simulink model "MPC_Kalman"  (R2015a)
settings: Solver=ode4  StartTime=0.0  StopTime=10  FixedStep=0.01  RelTol=1e-3
values from neighbouring files (symbols this model uses):
  delay_time = 0    [MPC-PID-Data-0ms.mat]    (also in MPC-PID-Data-150ms.mat = 0.15; MPC-PID-Data-250ms.mat = 0.25; MPC-PID-Data-50ms.mat = 0.05)
libraries: simulink x8
settings Model: Creator=LAB425  LastModifiedBy=LAB425

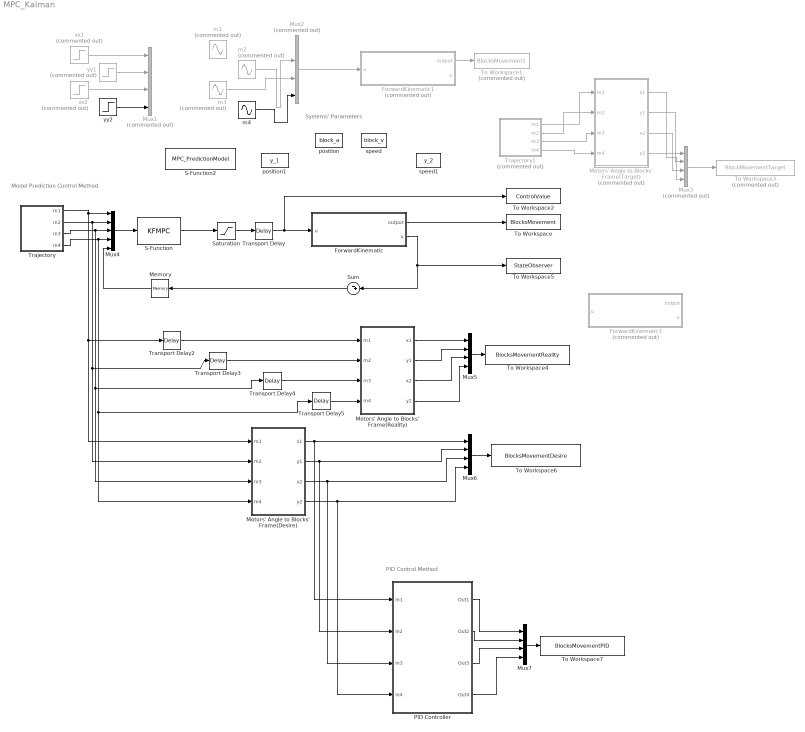
== system MPC_Kalman ==
  note: PID Control Method
  note: Model Prediction Control Method
  note: Systems' Parameters
  ForwardKinematic : MATLAB Function  TreatAsAtomicUnit=on
  ForwardKinematic1 : MATLAB Function  Commented=on  TreatAsAtomicUnit=on
  ForwardKinematic3 : MATLAB Function  Commented=on  TreatAsAtomicUnit=on
  Memory : Memory  X0=[0,0,0,0,0,0,0,0]
  Motors' Angle to Blocks' Frame(Desire) : MATLAB Function  TreatAsAtomicUnit=on
  Motors' Angle to Blocks' Frame(Reality) : MATLAB Function  TreatAsAtomicUnit=on
  "Motors' Angle to Blocks' Frame(Target) " : MATLAB Function  Commented=on  TreatAsAtomicUnit=on
  Mux1 : Mux  Commented=on
  Mux2 : Mux  Commented=on
  Mux3 : Mux  Commented=on
  Mux4 : Mux  Inputs=5
  Mux5 : Mux
  Mux6 : Mux
  Mux7 : Mux
  PID Controller : Subsystem
  S-Function : S-Function  FunctionName=KFMPC
  S-Function2 : S-Function  FunctionName=MPC_PredictionModel
  Saturation : Saturate  UpperLimit=1  LowerLimit=-1
  Sum : Sum  Inputs=-+|
  To Workspace : ToWorkspace  VariableName=BlocksMovement  SaveFormat=Timeseries  SampleTime=-1
  To Workspace1 : ToWorkspace  Commented=on  VariableName=BlocksMovement1  SaveFormat=Timeseries  SampleTime=-1
  To Workspace2 : ToWorkspace  VariableName=ControlValue  SaveFormat=Timeseries  SampleTime=-1
  To Workspace3 : ToWorkspace  Commented=on  VariableName=BlockMovementTarget  SaveFormat=Timeseries  SampleTime=-1
  To Workspace4 : ToWorkspace  VariableName=BlocksMovementReality  SaveFormat=Timeseries  SampleTime=-1
  To Workspace5 : ToWorkspace  VariableName=StateObserver  SaveFormat=Timeseries  SampleTime=-1
  To Workspace6 : ToWorkspace  VariableName=BlocksMovementDesire  SaveFormat=Timeseries  SampleTime=-1
  To Workspace7 : ToWorkspace  VariableName=BlocksMovementPID  SaveFormat=Timeseries  SampleTime=-1
  Trajectory : Subsystem
  Trajectory1 : Subsystem  Commented=on
  Transport Delay{,2..5} (5 alike) : TransportDelay  DelayTime=delay_time
  m1 : Sin  Commented=on  SampleTime=0
  m2 : Sin  Commented=on  Frequency=2  SampleTime=0
  m3 : Sin  Commented=on  Phase=3.14  SampleTime=0
  m4 : Sin  Frequency=2  Phase=3.14  SampleTime=0
  position : DataStoreMemory  DataStoreName=block_a  ReadBeforeWriteMsg=warning  WriteAfterWriteMsg=warning  WriteAfterReadMsg=warning  InitialValue=[0,0,0,0]  OutDataTypeStr=double
  position1 : DataStoreMemory  DataStoreName=y_1  ReadBeforeWriteMsg=warning  WriteAfterWriteMsg=warning  WriteAfterReadMsg=warning  InitialValue=[0,0,0,0]  OutDataTypeStr=double
  speed : DataStoreMemory  DataStoreName=block_v  ReadBeforeWriteMsg=warning  WriteAfterWriteMsg=warning  WriteAfterReadMsg=warning  InitialValue=[0,0,0,0]  OutDataTypeStr=double
  speed1 : DataStoreMemory  DataStoreName=y_2  ReadBeforeWriteMsg=warning  WriteAfterWriteMsg=warning  WriteAfterReadMsg=warning  InitialValue=[0,0,0,0]  OutDataTypeStr=double
  xx1 : Step  Commented=on  Time=0  Before=-2  After=-2
  xx2 : Step  Commented=on  Time=0  Before=0.5  After=0.5
  yy1 : Step  Commented=on  Time=0  Before=-2  After=-2
  yy2 : Step  Time=5  Before=1
  wires:
  xx1/1 -> Mux1/1
  yy2/1 -> Mux1/4
  yy1/1 -> Mux1/2
  xx2/1 -> Mux1/3
  m2/1 -> Mux2/2
  m3/1 -> Mux2/3
  m4/1 -> Mux2/4
  Mux2/1 -> ForwardKinematic1/1(u)
  ForwardKinematic1/1(output) -> To Workspace1/1
  Mux4/1 -> S-Function/1
  Memory/1 -> Mux4/5
  S-Function/1 -> Saturation/1
  Trajectory/1(m1) -> Motors' Angle to Blocks' Frame(Desire)/1(m1), Transport Delay2/1, Mux4/1
  Trajectory/3(m3) -> Motors' Angle to Blocks' Frame(Desire)/3(m3), Transport Delay4/1, Mux4/3
  Trajectory1/1(m1) -> "Motors' Angle to Blocks' Frame(Target) "/1(m1)
  Trajectory1/2(m2) -> "Motors' Angle to Blocks' Frame(Target) "/2(m2)
  Trajectory1/3(m3) -> "Motors' Angle to Blocks' Frame(Target) "/3(m3)
  Trajectory1/4(m4) -> "Motors' Angle to Blocks' Frame(Target) "/4(m4)
  Mux3/1 -> To Workspace3/1
  "Motors' Angle to Blocks' Frame(Target) "/1(x1) -> Mux3/1
  "Motors' Angle to Blocks' Frame(Target) "/2(y1) -> Mux3/2
  "Motors' Angle to Blocks' Frame(Target) "/3(x2) -> Mux3/3
  "Motors' Angle to Blocks' Frame(Target) "/4(y2) -> Mux3/4
  Trajectory/4(m4) -> Motors' Angle to Blocks' Frame(Desire)/4(m4), Transport Delay5/1, Mux4/4
  Motors' Angle to Blocks' Frame(Reality)/1(x1) -> Mux5/1
  Motors' Angle to Blocks' Frame(Reality)/2(y1) -> Mux5/2
  Motors' Angle to Blocks' Frame(Reality)/3(x2) -> Mux5/3
  Motors' Angle to Blocks' Frame(Reality)/4(y2) -> Mux5/4
  Mux5/1 -> To Workspace4/1
  Saturation/1 -> Transport Delay/1
  Sum/1 -> Memory/1
  Transport Delay2/1 -> Motors' Angle to Blocks' Frame(Reality)/1(m1)
  Transport Delay3/1 -> Motors' Angle to Blocks' Frame(Reality)/2(m2)
  Transport Delay4/1 -> Motors' Angle to Blocks' Frame(Reality)/3(m3)
  Transport Delay5/1 -> Motors' Angle to Blocks' Frame(Reality)/4(m4)
  ForwardKinematic/2(x) -> Sum/2, To Workspace5/1
  ForwardKinematic/1(output) -> To Workspace/1
  Transport Delay/1 -> ForwardKinematic/1(u), To Workspace2/1
  Mux6/1 -> To Workspace6/1
  Trajectory/2(m2) -> Motors' Angle to Blocks' Frame(Desire)/2(m2), Transport Delay3/1, Mux4/2
  Motors' Angle to Blocks' Frame(Desire)/1(x1) -> Mux6/1, PID Controller/1(in1)
  Motors' Angle to Blocks' Frame(Desire)/2(y1) -> Mux6/2, PID Controller/2(In2)
  Mux7/1 -> To Workspace7/1
  Motors' Angle to Blocks' Frame(Desire)/3(x2) -> Mux6/3, PID Controller/3(In3)
  Motors' Angle to Blocks' Frame(Desire)/4(y2) -> PID Controller/4(In4), Mux6/4
  PID Controller/1(Out1) -> Mux7/1
  PID Controller/2(Out2) -> Mux7/2
  PID Controller/3(Out3) -> Mux7/3
  PID Controller/4(Out4) -> Mux7/4

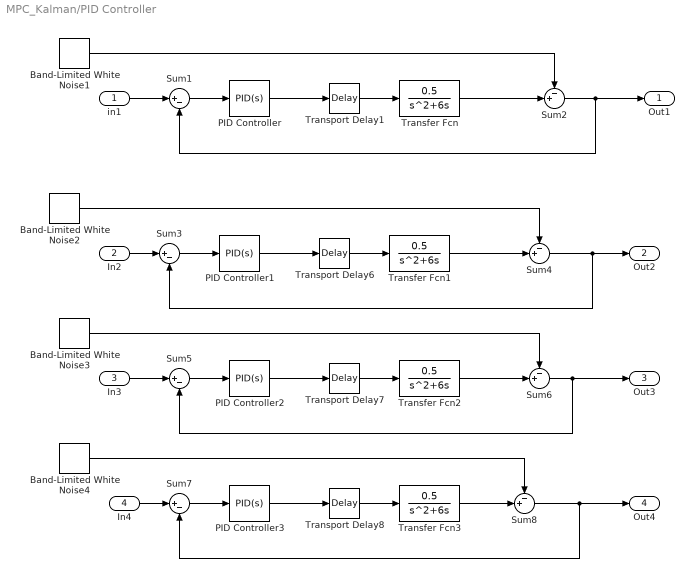
== system MPC_Kalman/PID Controller ==
  in1 : Inport
  In2 : Inport  Port=2
  In3 : Inport  Port=3
  In4 : Inport  Port=4
  Band-Limited White Noise{1..4} (4 alike) : simulink/Sources/Band-Limited White Noise  Cov=[0.00001]  Ts=0.01  seed=[23341]
  PID Controller{,1..3} (4 alike) : simulink/Continuous/PID Controller  Controller=PID  TimeDomain=Continuous-time  SampleTime=-1  IntegratorMethod=Forward Euler  FilterMethod=Forward Euler  Form=Parallel  UseFilter=on  ControllerParametersSource=internal  P=60  I=2  D=0  N=100  InitialConditionSource=internal  InitialConditionForIntegrator=0  InitialConditionForFilter=0  ExternalReset=none  LimitOutput=off  UpperSaturationLimit=inf  LowerSaturationLimit=-inf  LinearizeAsGain=on  AntiWindupMode=none  Kb=1  TrackingMode=off  Kt=1  PParamMin=[]  PParamMax=[]  IParamMin=[]  IParamMax=[]  DParamMin=[]  DParamMax=[]  NParamMin=[]  NParamMax=[]  KbParamMin=[]  KbParamMax=[]  KtParamMin=[]  KtParamMax=[]  POutMin=[]  POutMax=[]  IOutMin=[]  IOutMax=[]  DOutMin=[]  DOutMax=[]  NOutMin=[]  NOutMax=[]  KbOutMin=[]  KbOutMax=[]  KtOutMin=[]  KtOutMax=[]  IntegratorOutMin=[]  IntegratorOutMax=[]  FilterOutMin=[]  FilterOutMax=[]  SumOutMin=[]  SumOutMax=[]  SumI1OutMin=[]  SumI1OutMax=[]  SumI2OutMin=[]  SumI2OutMax=[]  SumI3OutMin=[]  SumI3OutMax=[]  SumDOutMin=[]  SumDOutMax=[]  SaturationOutMin=[]  SaturationOutMax=[]  IntegratorContinuousStateAttributes=''  IntegratorStateMustResolveToSignalObject=off  IntegratorRTWStateStorageClass=Auto  FilterContinuousStateAttributes=''  FilterStateMustResolveToSignalObject=off  FilterRTWStateStorageClass=Auto  DifferentiatorICPrevScaledInput=0  DifferentiatorOutMin=[]  DifferentiatorOutMax=[]
  Sum{1,3,5,7} (4 alike) : Sum  Inputs=|+-
  Sum{2,4,6,8} (4 alike) : Sum  Inputs=-+|
  Transfer Fcn{,1..3} (4 alike) : TransferFcn  Numerator=[0.5]  Denominator=[1 6 0]
  Transport Delay{1,6..8} (4 alike) : TransportDelay  DelayTime=delay_time
  Out1 : Outport
  Out2 : Outport  Port=2
  Out3 : Outport  Port=3
  Out4 : Outport  Port=4
  wires:
  Transport Delay1/1 -> Transfer Fcn/1
  PID Controller/1 -> Transport Delay1/1
  Sum1/1 -> PID Controller/1
  PID Controller2/1 -> Transport Delay7/1
  Transfer Fcn2/1 -> Sum6/2
  Sum5/1 -> PID Controller2/1
  Band-Limited White Noise3/1 -> Sum6/1
  Transport Delay7/1 -> Transfer Fcn2/1
  Transport Delay6/1 -> Transfer Fcn1/1
  Sum3/1 -> PID Controller1/1
  Transfer Fcn1/1 -> Sum4/2
  Band-Limited White Noise2/1 -> Sum4/1
  PID Controller1/1 -> Transport Delay6/1
  Sum2/1 -> Sum1/2, Out1/1
  Sum6/1 -> Sum5/2, Out3/1
  In2/1 -> Sum3/1
  Sum8/1 -> Sum7/2, Out4/1
  in1/1 -> Sum1/1
  In4/1 -> Sum7/1
  In3/1 -> Sum5/1
  PID Controller3/1 -> Transport Delay8/1
  Transfer Fcn3/1 -> Sum8/2
  Sum7/1 -> PID Controller3/1
  Band-Limited White Noise4/1 -> Sum8/1
  Transport Delay8/1 -> Transfer Fcn3/1
  Band-Limited White Noise1/1 -> Sum2/1
  Transfer Fcn/1 -> Sum2/2
  Sum4/1 -> Sum3/2, Out2/1

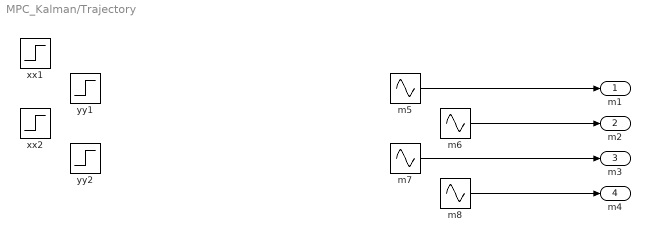
== system MPC_Kalman/Trajectory ==
  m5 : Sin  SampleTime=0
  m6 : Sin  Frequency=2  SampleTime=0
  m7 : Sin  Phase=3.14  SampleTime=0
  m8 : Sin  Frequency=2  Phase=3.14  SampleTime=0
  xx1 : Step
  xx2 : Step  After=-1
  yy1 : Step
  yy2 : Step  After=-1
  m1 : Outport
  m2 : Outport  Port=2
  m3 : Outport  Port=3
  m4 : Outport  Port=4
  wires:
  m6/1 -> m2/1
  m5/1 -> m1/1
  m7/1 -> m3/1
  m8/1 -> m4/1

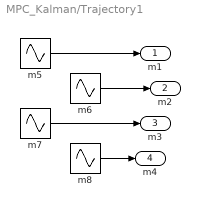
== system MPC_Kalman/Trajectory1 ==
  m5 : Sin  SampleTime=0
  m6 : Sin  Frequency=2  SampleTime=0
  m7 : Sin  Phase=3.14  SampleTime=0
  m8 : Sin  Frequency=2  Phase=3.14  SampleTime=0
  m1 : Outport
  m2 : Outport  Port=2
  m3 : Outport  Port=3
  m4 : Outport  Port=4
  wires:
  m6/1 -> m2/1
  m5/1 -> m1/1
  m7/1 -> m3/1
  m8/1 -> m4/1

== matlab function MPC_Kalman/ForwardKinematic1 ==
  data: output output; u input; block_v data_store_memory; block_a data_store_memory; x output
function [output,x] = RobotForwardKinematic(u) %输入1x4
global block_v block_a 
%block_v：上一时刻的角速度
%block_a：上一时刻的角度
%% 单电机状态方程
A = [0 1 0 0 0 0 0 0;
     0.005 0.045 0 0 0 0 0 0;
     0 0 0 1 0 0 0 0;
     0 0 0.0185 0.0251 0 0 0 0;
     0 0 0 0 0 1 0 0;
     0 0 0 0 0.0065 -0.0258 0 0;
     0 0 0 0 0 0 0 1;
     0 0 0 0 0 0 -0.023 0.0084]; 
b = [0 0 0 0;
     1.8899 0 0 0;
     0 0 0 0;
     0 1.8777 0 0;
     0 0 0 0;
     0 0 1.7655 0;
     0 0 0 0;
     0 0 0 1.7735];
C = [0 1 0 0 0 0 0 0;
     0 0 0 1 0 0 0 0;
     0 0 0 0 0 1 0 0;
     0 0 0 0 0 0 0 1];
% X = [0,1;-a2,-a1];
% H = [0,b]';
% C = [0,1];
delta_u = u - block_a;
v = delta_u ./ 0.01;
a = (v - block_v) ./ 0.01;
block_v = v;
block_a = u;
x = [v(1);a(1);v(2);a(2);v(3);a(3);v(4);a(4)];
output = C * (A * x + b * u);
%%

== matlab function MPC_Kalman/Motors' Angle to Blocks' Frame(Reality) ==
  data: x1 output; m1 input; y1 output; x2 output; m2 input; m3 input; m4 input; y2 output
function [x1,y1,x2,y2] = Signal(m1,m2,m3,m4)



%m1,m2,m3,m4为四个电机的当前时刻的角度值

%最远距离
D = 1.8;
% %螺距
% n = 0.02;
% %最大圈数
% ratio = D / n;
v=sqrt(0.01)*randn(4,1);
x1 = m1 * D + v(1);
y1 = m2 * D + v(2);
x2 = m3 * D + v(3);
y2 = m4 * D + v(4);

if x1>=2
    x1=2;
else
    if x1<=-2
        x1=-2;
    end
end
if x2>=2
    x2=2;
else
    if x2<=-2
        x2=-2;
    end
end
if y1>=2
    y1=2;
else
    if y1<=-2
        y1=-2;
    end
end
if y2>=2
    y2=2;
else
    if y2<=-2
        y2=-2;
    end
end

== matlab function MPC_Kalman/Motors' Angle to Blocks' Frame(Desire) ==
  data: x1 output; m1 input; y1 output; x2 output; m2 input; m3 input; m4 input; y2 output
function [x1,y1,x2,y2] = Signal(m1,m2,m3,m4)



%m1,m2,m3,m4为四个电机的当前时刻的角度值

%最远距离
D = 1.85;
% %螺距
% n = 0.02;
% %最大圈数
% ratio = D / n;
v=sqrt(0.01)*randn(4,1);
x1 = m1 * D;
y1 = m2 * D;
x2 = m3 * D;
y2 = m4 * D;

if x1>=2
    x1=2;
else
    if x1<=-2
        x1=-2;
    end
end
if x2>=2
    x2=2;
else
    if x2<=-2
        x2=-2;
    end
end
if y1>=2
    y1=2;
else
    if y1<=-2
        y1=-2;
    end
end
if y2>=2
    y2=2;
else
    if y2<=-2
        y2=-2;
    end
end

== matlab function MPC_Kalman/ForwardKinematic ==
  data: output output; u input; block_v data_store_memory; block_a data_store_memory; x output; y_1 data_store_memory; y_2 data_store_memory
function [output,x] = RobotForwardKinematic(u) %输入1x4
global y_1 y_2
%block_v：上一时刻的角速度
%block_a：上一时刻的角度
%% 单电机状态方程
A = [0 1 0 0 0 0 0 0;
     0.005 0.045 0 0 0 0 0 0;
     0 0 0 1 0 0 0 0;
     0 0 0.0185 0.0251 0 0 0 0;
     0 0 0 0 0 1 0 0;
     0 0 0 0 0.0065 -0.0258 0 0;
     0 0 0 0 0 0 0 1;
     0 0 0 0 0 0 -0.023 0.0084]; %8x8
b = [0 0 0 0;
     1.8899 0 0 0;
     0 0 0 0;
     0 1.8777 0 0;
     0 0 0 0;
     0 0 1.7655 0;
     0 0 0 0;
     0 0 0 1.7735]; % 8x4
C = [0 1 0 0 0 0 0 0;
     0 0 0 1 0 0 0 0;
     0 0 0 0 0 1 0 0;
     0 0 0 0 0 0 0 1];
% X = [0,1;-a2,-a1];
% H = [0,b]';
% C = [0,1];

% delta_u = u - block_a;
% v = delta_u ./ 0.01;
% a = (v - block_v) ./ 0.01;
% block_v = v;
% block_a = u;
% x = [v(1);a(1);v(2);a(2);v(3);a(3);v(4);a(4)];

y = [y_2(1);y_1(1);y_2(2);y_1(2);y_2(3);y_1(3);y_2(4);y_1(4)];
x = y;
v=sqrt(0.001)*randn(4,1);
output = C * (A * x + b * u) + v;
y_2 = y_1;
y_1 = output;

%%
% %最远距离
% D = 1.8;
% % %螺距
% % n = 0.02;
% % %最大圈数
% % ratio = D / n;
% v=sqrt(0.01)*randn(4,1);
% x1 = u(1) * D + v(1);
% y1 = u(2) * D + v(2);
% x2 = u(3) * D + v(3);
% y2 = u(4) * D + v(4);
% 
% if x1>=2
%     x1=2;
% else
%     if x1<=-2
%         x1=-2;
%     end
% end
% if x2>=2
%     x2=2;
% else
%     if x2<=-2
%         x2=-2;
%     end
% end
% if y1>=2
%     y1=2;
% else
%     if y1<=-2
%         y1=-2;
%     end
% end
% if y2>=2
%     y2=2;
% else
%     if y2<=-2
%         y2=-2;
%     end
% end
% output = [x1;y1;x2;y2];
% y_2 = y_1;
% y_1 = output;
% y = [y_2(1);y_1(1);y_2(2);y_1(2);y_2(3);y_1(3);y_2(4);y_1(4)];
% x = y;
%

== matlab function MPC_Kalman/Motors' Angle to Blocks' Frame(Target)  ==
  data: x1 output; m1 input; y1 output; x2 output; m2 input; m3 input; m4 input; y2 output
function [x1,y1,x2,y2] = Signal(m1,m2,m3,m4)



%m1,m2,m3,m4为四个电机的当前时刻的角度值

%最远距离
D = 1.8;
% %螺距
% n = 0.02;
% %最大圈数
% ratio = D / n;
v=sqrt(0.01)*randn(4,1);
x1 = m1 * D;
y1 = m2 * D;
x2 = m3 * D;
y2 = m4 * D;

if x1>=2
    x1=2;
else
    if x1<=-2
        x1=-2;
    end
end
if x2>=2
    x2=2;
else
    if x2<=-2
        x2=-2;
    end
end
if y1>=2
    y1=2;
else
    if y1<=-2
        y1=-2;
    end
end
if y2>=2
    y2=2;
else
    if y2<=-2
        y2=-2;
    end
end

== matlab function MPC_Kalman/ForwardKinematic3 ==
  data: output output; u input; block_v data_store_memory; block_a data_store_memory; x output
function [output,x] = RobotForwardKinematic(u) %输入1x4
global block_v block_a 
%block_v：上一时刻的角速度
%block_a：上一时刻的角度
%% 单电机状态方程
A = [0 1 0 0 0 0 0 0;
     0.0049 0.0445 0 0 0 0 0 0;
     0 0 0 1 0 0 0 0;
     0 0 0.018 0.025 0 0 0 0;
     0 0 0 0 0 1 0 0;
     0 0 0 0 0.0063 -0.026 0 0;
     0 0 0 0 0 0 0 1;
     0 0 0 0 0 0 -0.0225 0.0087]; %8x8
b = [0 0 0 0;
     1.889 0 0 0;
     0 0 0 0;
     0 1.876 0 0;
     0 0 0 0;
     0 0 1.765 0;
     0 0 0 0;
     0 0 0 1.775]; % 8x4
C = [0 1 0 0 0 0 0 0;
     0 0 0 1 0 0 0 0;
     0 0 0 0 0 1 0 0;
     0 0 0 0 0 0 0 1];
% X = [0,1;-a2,-a1];
% H = [0,b]';
% C = [0,1];
% delta_u = u - block_a;
% v = delta_u ./ 0.01;
% a = (v - block_v) ./ 0.01;
% block_v = v;
% block_a = u;
x = [v(1);a(1);v(2);a(2);v(3);a(3);v(4);a(4)];
output = C * (A * x + b * u);
%%
